simulink model "bola_saltitonaP41"  (R2015a)
settings: Solver=ode3  StartTime=0.0  StopTime=13  FixedStep=1e-4  RelTol=1e-3
libraries: simulink x2
settings Model: Creator=ModSim  LastModifiedBy=João Santos
settings DataIOCC: InspectSignalLogs=on
settings DebuggingCC: MaxConsecutiveZCsMsg=none

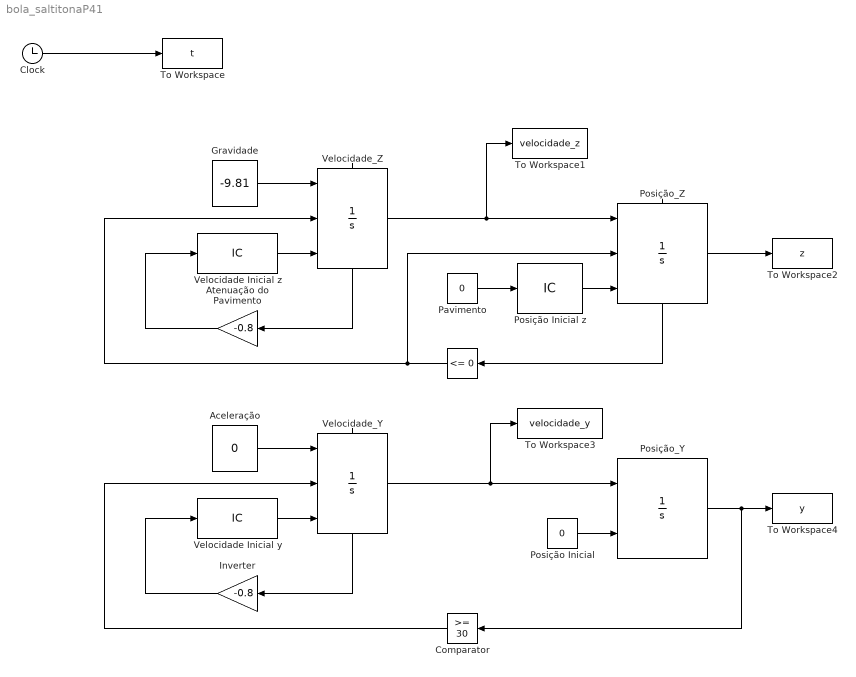
== system bola_saltitonaP41 ==
  " " : simulink/Logic and Bit Operations/Compare To Zero  relop=<=  OutDataTypeStr=boolean
  " Posição_Y" : Integrator  InitialConditionSource=external  LimitOutput=on
  " Posição_Z" : Integrator  ExternalReset=rising  InitialConditionSource=external  LimitOutput=on  LowerSaturationLimit=0  ShowStatePort=on
  Aceleração : Constant  Value=0
  Atenuação do Pavimento : Gain  Gain=-0.8
  Clock : Clock
  Comparator : simulink/Logic and Bit Operations/Compare To Constant  relop=>=  const=30  OutDataTypeStr=boolean
  Gravidade : Constant  Value=-9.81
  Inverter : Gain  Gain=-0.8
  Pavimento : Constant  Value=0
  Posição Inicial : Constant  Value=0
  Posição Inicial z : InitialCondition  Value=10
  To Workspace : ToWorkspace  VariableName=t  SampleTime=-1
  To Workspace1 : ToWorkspace  VariableName=velocidade_z  SampleTime=-1
  To Workspace2 : ToWorkspace  VariableName=z  SampleTime=-1
  To Workspace3 : ToWorkspace  VariableName=velocidade_y  SampleTime=-1
  To Workspace4 : ToWorkspace  VariableName=y  SampleTime=-1
  Velocidade Inicial y : InitialCondition  Value=5
  Velocidade Inicial z : InitialCondition  Value=0
  Velocidade_Y : Integrator  ExternalReset=rising  InitialConditionSource=external  ShowStatePort=on
  Velocidade_Z : Integrator  ExternalReset=rising  InitialConditionSource=external  ShowStatePort=on
  wires:
  Velocidade Inicial z/1 -> Velocidade_Z/3
  " "/1 -> Velocidade_Z/2, " Posição_Z"/2
  Clock/1 -> To Workspace/1
  Posição Inicial z/1 -> " Posição_Z"/3
  Pavimento/1 -> Posição Inicial z/1
  " Posição_Z"/1 -> To Workspace2/1
  Velocidade_Z/1 -> " Posição_Z"/1, To Workspace1/1
  Gravidade/1 -> Velocidade_Z/1
  " Posição_Z"/State -> " "/1
  Velocidade_Z/State -> Atenuação do Pavimento/1
  Atenuação do Pavimento/1 -> Velocidade Inicial z/1
  Velocidade_Y/1 -> " Posição_Y"/1, To Workspace3/1
  Comparator/1 -> Velocidade_Y/2
  Aceleração/1 -> Velocidade_Y/1
  Velocidade Inicial y/1 -> Velocidade_Y/3
  " Posição_Y"/1 -> Comparator/1, To Workspace4/1
  Velocidade_Y/State -> Inverter/1
  Inverter/1 -> Velocidade Inicial y/1
  Posição Inicial/1 -> " Posição_Y"/2
